simulink model "dummy2"  (R2020a)
settings: Solver=VariableStepAuto  StartTime=0.0  StopTime=10.0  RelTol=1e-3
settings Model: Creator=dhruv  LastModifiedBy=dhruv

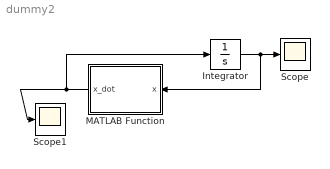
== system dummy2 ==
  Integrator : Integrator  InitialCondition=10
  MATLAB Function : MATLAB Function  TreatAsAtomicUnit=on
  Scope : Scope
  Scope1 : Scope
  wires:
  Integrator/1 -> Scope/1, MATLAB Function/1(x)
  MATLAB Function/1(x_dot) -> Integrator/1, Scope1/1

== matlab function dummy2/MATLAB Function ==
  data: x input; x_dot output
function x_dot = fcn(x)

x_dot = x;
